simulink model "lab0_Simulation_PID_Controller_Design"  (R2020b)
settings: Solver=VariableStepAuto  StartTime=0.0  StopTime=1  RelTol=1e-3
InitFcn:
  | PID_Controller_Design
undefined symbols (not defined in the file): K_D, K_I, K_P, sens, T_L
settings Model: Creator=Davide  LastModifiedBy=Musta
settings SolverCC: ZeroCrossAlgorithm=Adaptive
settings DebuggingCC: IgnoredZcDiagnostic=none

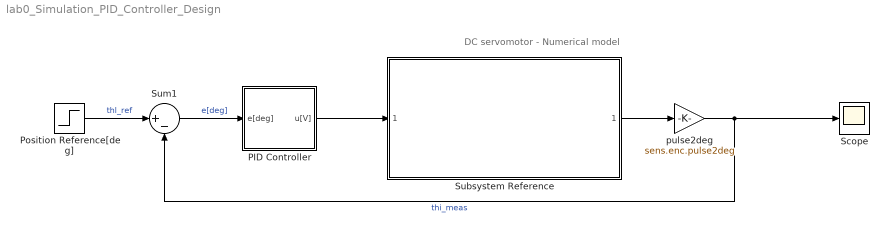
== system lab0_Simulation_PID_Controller_Design ==
  note: DC servomotor - Numerical model
  PID Controller : Subsystem
  Position Reference[deg] : Step  Time=0  After=10  SampleTime=0
  Scope : Scope
  Subsystem Reference : Subsystem  ReferencedSubsystem=plant_Model
  Sum1 : Sum  Inputs=|+-
  pulse2deg : Gain  Gain=sens.enc.pulse2deg
  wires:
  Position Reference[deg]/1 -> Sum1/1  "thl_ref"
  Sum1/1 -> PID Controller/1(e[deg])  "e[deg]"
  PID Controller/1(u[V]) -> Subsystem Reference/1
  Subsystem Reference/1 -> pulse2deg/1
  pulse2deg/1 -> Sum1/2, Scope/1  "thi_meas"

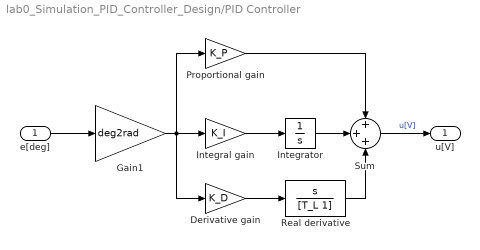
== system lab0_Simulation_PID_Controller_Design/PID Controller ==
  e[deg] : Inport
  Derivative gain : Gain  Gain=K_D
  Gain1 : Gain  Gain=deg2rad
  Integral gain : Gain  Gain=K_I
  Integrator : Integrator
  Proportional gain : Gain  Gain=K_P
  Real derivative : TransferFcn  Numerator=[1 0]  Denominator=[T_L 1]
  Sum : Sum  Inputs=+++
  u[V] : Outport
  wires:
  e[deg]/1 -> Gain1/1
  Integrator/1 -> Sum/2
  Gain1/1 -> Proportional gain/1, Derivative gain/1, Integral gain/1
  Proportional gain/1 -> Sum/1
  Derivative gain/1 -> Real derivative/1
  Real derivative/1 -> Sum/3
  Integral gain/1 -> Integrator/1
  Sum/1 -> u[V]/1  "u[V]"
